simulink model "TestSTARC_ABL_possible_simp"  (R2017a)
settings: Solver=FixedStepDiscrete  StartTime=0.0  StopTime=10  FixedStep=0.015  RelTol=1e-3  EnableMultiTasking=on
libraries: Lib_Turbo_PGenerator_TMATS x2, Lib_PF_LineDC_TMATS x1, Lib_PF_BusLoadDC_TMATS x1, Lib_Solve_SSNRSolverJC_TMATS x1, Lib_PF_BusSlackDC_TMATS x1
settings Model: Creator=jwchapm2  LastModifiedBy=glthoma1
settings DataIOCC: LimitDataPoints=on  SaveFormat=Array
settings OptimizationCC: LifeSpan=inf
settings DebuggingCC: SFUnexpectedBacktrackingDiag=warning  SFNoUnconditionalDefaultTransitionDiag=warning  SFExecutionAtInitializationDiag=none
settings HardwareCC: ProdBitPerPointer=32  ProdBitPerSizeT=32  ProdBitPerPtrDiffT=32  ProdLargestAtomicFloat=None  ProdIntDivRoundTo=Undefined  ProdEndianess=Unspecified  ProdWordSize=32  ProdHWDeviceType=32-bit Generic
settings ModelReferenceCC: PropagateSignalLabelsOutOfModel=off
settings GRTTargetCC: TargetLangStandard=C89/C90 (ANSI)  GeneratePreprocessorConditionals=Disable all
settings ConfigComp: CovMetricSettings=dw  CovHtmlReporting=on  CovSaveCumulativeToWorkspaceVar=on  CovSaveSingleToWorkspaceVar=on  CovExternalEMLEnable=off

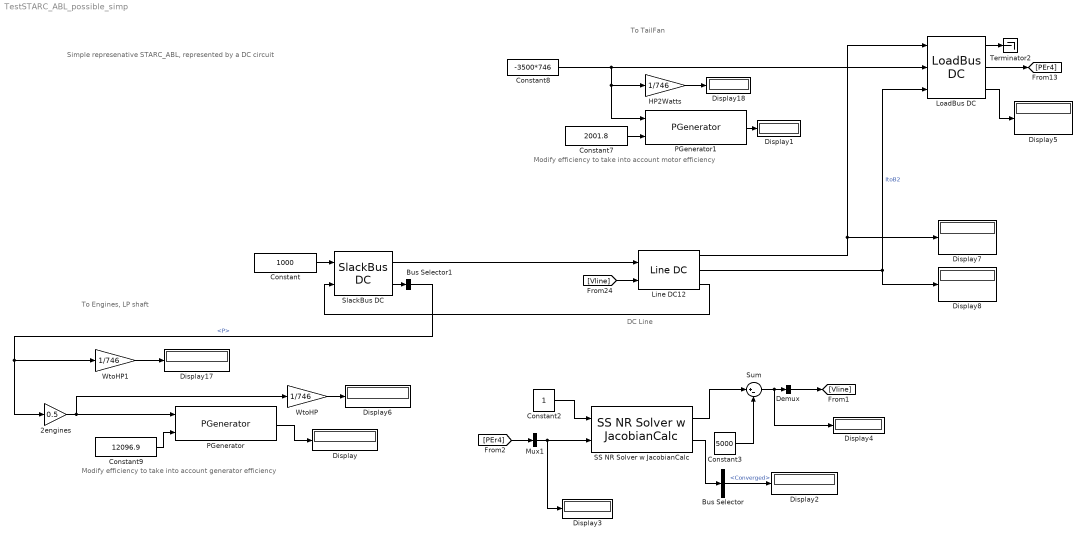
== system TestSTARC_ABL_possible_simp ==
  note: To Engines, LP shaft
  note: To TailFan
  note: DC Line
  note: Modify efficiency to take into
      | account generator efficiency
  note: Modify efficiency to take into
      | account motor efficiency
  note: Simple represenative STARC_ABL,
      | represented by a DC circuit
  2engines : Gain  Gain=0.5
  Bus Selector : BusSelector  OutputSignals=Converged
  Bus Selector1 : BusSelector  OutputSignals=P
  Constant : Constant  Value=1000
  Constant2 : Constant
  Constant3 : Constant  Value=5000
  Constant7 : Constant  Value=2001.8
  Constant8 : Constant  Value=-3500*746
  Constant9 : Constant  Value=12096.9
  Demux : Demux  Outputs=1
  Display{,1..8,17..18} (11 alike) : Display
  HP2Watts : Gain  Gain=1/746
  Line DC12 : Lib_PF_LineDC_TMATS/Line DC  R_M=0.01
  LoadBus DC : Lib_PF_BusLoadDC_TMATS/LoadBus DC  PeInEN_M=on  P_M=-2  BlkNm_M=double(gcb)
  Mux1 : Mux  Inputs=1
  PGenerator : Lib_Turbo_PGenerator_TMATS/PGenerator  Eff_M=0.99
  PGenerator1 : Lib_Turbo_PGenerator_TMATS/PGenerator  Eff_M=1.01
  SS NR Solver w JacobianCalc : Lib_Solve_SSNRSolverJC_TMATS/SS NR Solver w JacobianCalc  SJac_Per_M=[0.00001]  SNR_IC_M=[973]+5000  SNR_DX_M=5  SNR_Mx_M=100000  SNR_Mn_M=0.000001  SJacobianAttempts_M=20  Cond_Limits_M=1e-7
  SlackBus DC : Lib_PF_BusSlackDC_TMATS/SlackBus DC
  Sum : Sum  Inputs=|+-
  Terminator2 : Terminator
  WtoHP : Gain  Gain=1/746
  WtoHP1 : Gain  Gain=1/746
  wires:
  Constant/1 -> SlackBus DC/1
  Constant2/1 -> SS NR Solver w JacobianCalc/1
  SS NR Solver w JacobianCalc/1 -> Sum/1
  Mux1/1 -> Display3/1, SS NR Solver w JacobianCalc/2
  Sum/1 -> Display4/1, Demux/1
  Constant3/1 -> Sum/2
  SS NR Solver w JacobianCalc/2 -> Bus Selector/1
  Bus Selector/1 -> Display2/1  "<Converged>"
  Line DC12/3 -> SlackBus DC/2
  LoadBus DC/2 -> [PEr4]
  [Vline] -> Line DC12/2
  Demux/1 -> [Vline]
  [PEr4] -> Mux1/1
  SlackBus DC/2 -> Bus Selector1/1
  Constant7/1 -> PGenerator1/2
  PGenerator/1 -> Display/1
  Bus Selector1/1 -> WtoHP1/1, 2engines/1  "<P>"
  2engines/1 -> WtoHP/1, PGenerator/1
  SlackBus DC/1 -> Line DC12/1
  WtoHP/1 -> Display6/1
  WtoHP1/1 -> Display17/1
  HP2Watts/1 -> Display18/1
  Constant8/1 -> LoadBus DC/2, PGenerator1/1, HP2Watts/1
  Constant9/1 -> PGenerator/2
  LoadBus DC/3 -> Display5/1
  PGenerator1/1 -> Display1/1
  Line DC12/2 -> LoadBus DC/3, Display8/1  "ItoB2"
  Line DC12/1 -> LoadBus DC/1, Display7/1
  LoadBus DC/1 -> Terminator2/1
